simulink model "homework5_1"  (R2021a)
settings: Solver=VariableStepAuto  StartTime=0.0  StopTime=16  RelTol=1e-3
settings Model: Creator=Godfly  LastModifiedBy=Godfly
settings OptimizationCC: BooleanDataType=off

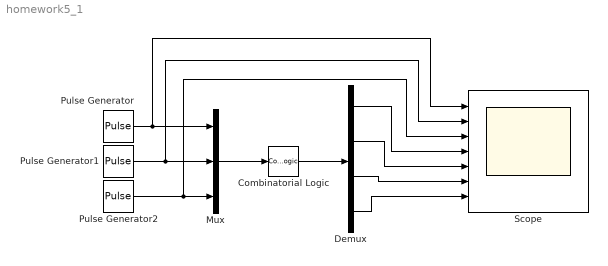
== system homework5_1 ==
  Combinatorial Logic : CombinatorialLogic  TruthTable=[1 1 1 1; 1 0 1 0; 1 0 1 0; 1 0 1 0; 1 0 1 0; 1 0 1 0; 1 0 1 0; 0 1 1 0]
  Demux : Demux
  Mux : Mux  Inputs=3
  Pulse Generator : DiscretePulseGenerator  PulseType=Time based  PulseWidth=50  PhaseDelay=1
  Pulse Generator1 : DiscretePulseGenerator  PulseType=Time based  Period=4  PulseWidth=50  PhaseDelay=2
  Pulse Generator2 : DiscretePulseGenerator  PulseType=Time based  Period=8  PulseWidth=50  PhaseDelay=4
  Scope : Scope  NumInputPorts=7
  wires:
  Mux/1 -> Combinatorial Logic/1
  Combinatorial Logic/1 -> Demux/1
  Pulse Generator/1 -> Scope/1, Mux/1
  Pulse Generator1/1 -> Scope/2, Mux/2
  Pulse Generator2/1 -> Scope/3, Mux/3
  Demux/1 -> Scope/4
  Demux/2 -> Scope/5
  Demux/3 -> Scope/6
  Demux/4 -> Scope/7
